simulink model "auv_full_system_decomposed"  (R2026a)
settings: Solver=FixedStepDiscrete  StopTime=90  FixedStep=0.0125
undefined symbols (not defined in the file or in its folder): DiscIntNeverNeededParam
settings Model: Creator=muthuraam  LastModifiedBy=muthuraam

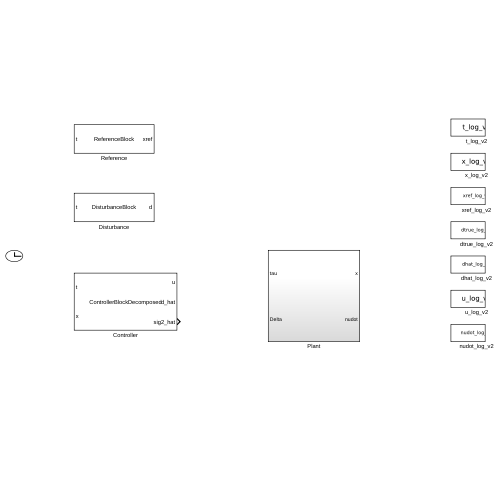
[thumbnail: Simulink's stored preview of the top-level diagram]
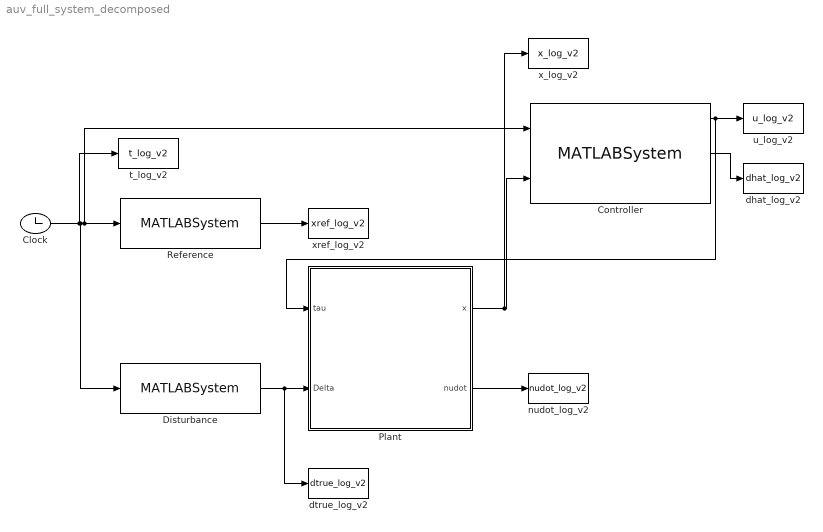
== system auv_full_system_decomposed ==
  Clock : Clock
  Controller : MATLABSystem  System=ControllerBlockDecomposed  SimulateUsing=Interpreted execution
      mask Type: ControllerBlockDecomposed
  Disturbance : MATLABSystem  System=DisturbanceBlock  SimulateUsing=Interpreted execution
      mask Type: DisturbanceBlock
  Plant : Subsystem
  Reference : MATLABSystem  System=ReferenceBlock  SimulateUsing=Interpreted execution
      mask Type: ReferenceBlock
  dhat_log_v2 : ToWorkspace  VariableName=dhat_log_v2  SampleTime=-1
  dtrue_log_v2 : ToWorkspace  VariableName=dtrue_log_v2  SampleTime=-1
  nudot_log_v2 : ToWorkspace  VariableName=nudot_log_v2  SampleTime=-1
  t_log_v2 : ToWorkspace  VariableName=t_log_v2  SampleTime=-1
  u_log_v2 : ToWorkspace  VariableName=u_log_v2  SampleTime=-1
  x_log_v2 : ToWorkspace  VariableName=x_log_v2  SampleTime=-1
  xref_log_v2 : ToWorkspace  VariableName=xref_log_v2  SampleTime=-1
  wires:
  Controller/2 -> dhat_log_v2/1
  Controller/1 -> u_log_v2/1, Plant/1(tau)
  Plant/2(nudot) -> nudot_log_v2/1
  Reference/1 -> xref_log_v2/1
  Plant/1(x) -> x_log_v2/1, Controller/2
  Disturbance/1 -> dtrue_log_v2/1, Plant/2(Delta)
  Clock/1 -> Reference/1, Controller/1, Disturbance/1, t_log_v2/1

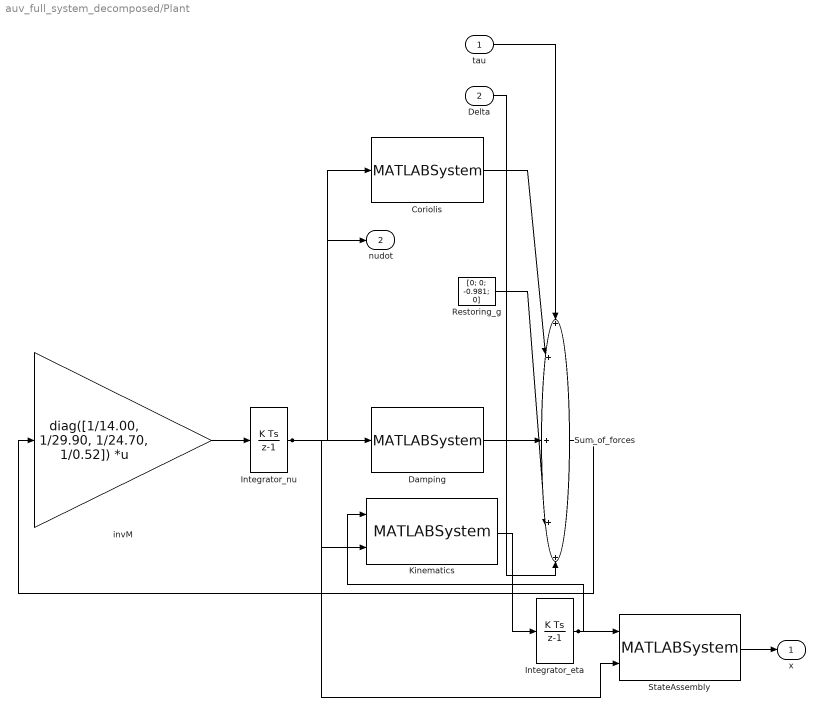
== system auv_full_system_decomposed/Plant ==
  tau : Inport
  Delta : Inport  Port=2
  Coriolis : MATLABSystem  System=CoriolisBlock  SimulateUsing=Interpreted execution
      mask Type: CoriolisBlock
  Damping : MATLABSystem  System=DampingBlock  SimulateUsing=Interpreted execution
      mask Type: DampingBlock
  Integrator_eta : DiscreteIntegrator  SampleTime=-1  ICPrevOutput=DiscIntNeverNeededParam  ICPrevScaledInput=DiscIntNeverNeededParam
  Integrator_nu : DiscreteIntegrator  SampleTime=-1  ICPrevOutput=DiscIntNeverNeededParam  ICPrevScaledInput=DiscIntNeverNeededParam
  Kinematics : MATLABSystem  System=KinematicsBlock  SimulateUsing=Interpreted execution
      mask Type: KinematicsBlock
  Restoring_g : Constant  Value=[0; 0; -0.981; 0]
  StateAssembly : MATLABSystem  System=StateAssemblyBlock  SimulateUsing=Interpreted execution
      mask Type: StateAssemblyBlock
  Sum_of_forces : Sum  Inputs=+++++
  invM : Gain  Gain=diag([1/14.00, 1/29.90, 1/24.70, 1/0.52])  Multiplication=Matrix(K*u)
  x : Outport
  nudot : Outport  Port=2
  wires:
  Integrator_eta/1 -> StateAssembly/1, Kinematics/1
  Kinematics/1 -> Integrator_eta/1
  Coriolis/1 -> Sum_of_forces/2
  Damping/1 -> Sum_of_forces/3
  Delta/1 -> Sum_of_forces/5
  Sum_of_forces/1 -> invM/1
  tau/1 -> Sum_of_forces/1
  Restoring_g/1 -> Sum_of_forces/4
  Integrator_nu/1 -> Kinematics/2, nudot/1, Damping/1, Coriolis/1, StateAssembly/2
  StateAssembly/1 -> x/1
  invM/1 -> Integrator_nu/1
